simulink library "lib_EMachine_2017a"  (R2017b)
settings: Solver=VariableStepAuto  StartTime=0.0  StopTime=10.0  RelTol=1e-3
undefined symbols (not defined in the file): EngineTorqueReal, mot, motor_Trq, t_amb, time, tloop
libraries: simulink x5, autolibmappedmotor x3
(part 1 of 3)
settings Model: Creator=Di Russo  LastModifiedBy=Lyu19
settings CodeAppCC: StateflowObjectComments=on

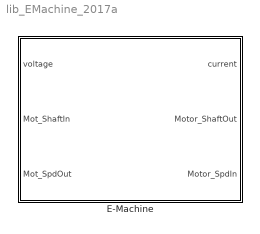
== system lib_EMachine_2017a ==
  E-Machine : Subsystem
      mask Display:
      | image('Images/motor.png')
      | color('red');
      | port_label('Input',1,'Volt');
      | port_label('Input',2,'ShaftIn');
      | port_label('Input',3,'SpdOut');
      | port_label('Output',1,'Crr');
      | port_label('Output',2,'ShaftOut');
      | port_label('Output',3,'SpdIn');

== system lib_EMachine_2017a/E-Machine ==
  voltage : Inport
  Mot_ShaftIn : Inport  Port=2
  Mot_SpdOut : Inport  Port=3
  Clutch Temporary 1 : Subsystem  Commented=on
  IMG Plant : Subsystem
      mask Display:
      | image('Images\Motor.png')
      | color('red');
      | port_label('Input',2,'Volt');
      | port_label('Input',3,'ShaftIn');
      | port_label('Input',4,'SpdOut');
      | port_label('Output',2,'Crr');
      | port_label('Output',3,'ShaftOut');
      | port_label('Output',4,'SpdIn');
  IMG Plant2 : Subsystem  Commented=on
      mask Display:
      | image('Images/motor.png')
      | color('red');
      | port_label('Input',2,'Volt');
      | port_label('Input',3,'SpdOut');
      | port_label('Input',1,'MCU_cmd');
      | port_label('Input',4,'ShaftIn');
      | port_label('Output',1,'Sensor_Out');
      | port_label('Output',2,'Crr');
      | port_label('Output',3,'MotTrqOut');
      | port_label('Output',4,'MotSpdIn');
  Soft MCU : Subsystem
      mask Display: image('SoftECU.jpg')
  current : Outport
  Motor_ShaftOut : Outport  Port=2
  Motor_SpdIn : Outport  Port=3
  tag scope: MCU_to_HCU=global
  wires:
  IMG Plant/4(SpdIn) -> Motor_SpdIn/1
  Mot_SpdOut/1 -> IMG Plant/4(SpdOut)
  Soft MCU/1(Out) -> [MCU_to_HCU]
  Soft MCU/2(Out1) -> IMG Plant/1("In1 ")  "MCU_to_Actuators"
  [HCU_to_HV_CAN] -> Soft MCU/1(In)
  IMG Plant/1(Out1) -> Soft MCU/2(In1)  "Sensors_to_MCU"
  Mot_ShaftIn/1 -> IMG Plant/3(MotShaftIn)
  IMG Plant/3(MotShaftOut) -> Motor_ShaftOut/1
  voltage/1 -> IMG Plant/2(voltage)
  IMG Plant/2(current) -> current/1

== system lib_EMachine_2017a/E-Machine/Clutch Temporary 1 ==
  In1 : Inport
  Constant : Constant  Value=0
  Memory : Memory
  Saturation : Saturate  UpperLimit=inf  LowerLimit=0
  Switch : Switch  Criteria=u2 > Threshold
  Out1 : Outport
  wires:
  Saturation/1 -> Memory/1
  Memory/1 -> Switch/1
  Constant/1 -> Switch/3
  In1/1 -> Saturation/1
  [cltch] -> Switch/2
  Switch/1 -> Out1/1

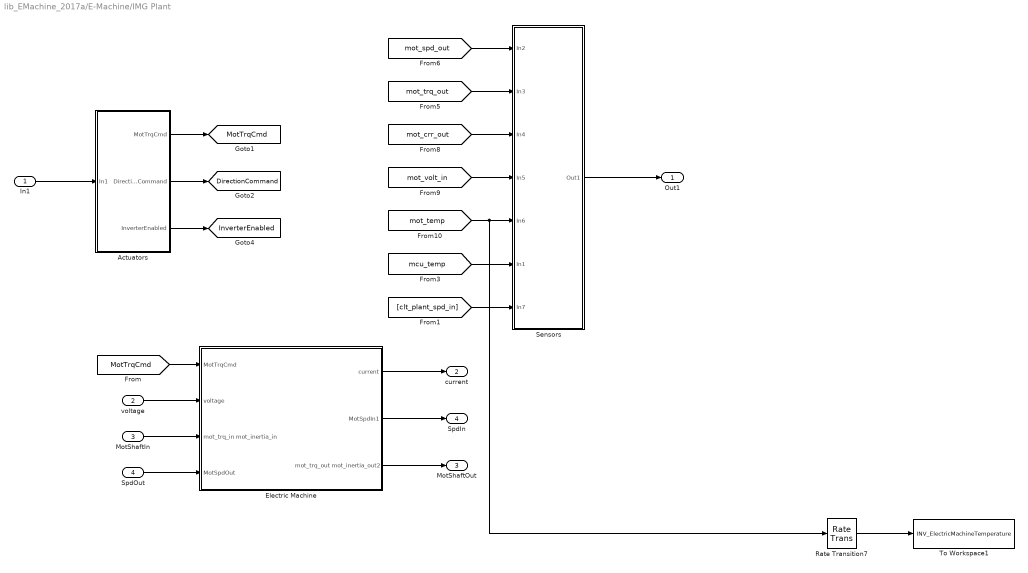
== system lib_EMachine_2017a/E-Machine/IMG Plant ==
  "In1 " : Inport
  voltage : Inport  Port=2
  MotShaftIn : Inport  Port=3
  SpdOut : Inport  Port=4
  " Actuators" : Subsystem
  Electric Machine : Subsystem
      mask Display:
      | image('Images\Motor.png')
      | color('red');
      | port_label('Input',1,'MotTrqCmd');
      | port_label('Input',2,'Volt');
      | port_label('Input',3,'ShaftIn');
      | port_label('Input',4,'SpdOut');
      | port_label('Output',1,'Crr')
      | port_label('Output',2,'SpdIn')
  Rate Transition7 : RateTransition  OutPortSampleTime=1
  Sensors : Subsystem
  To Workspace1 : ToWorkspace  VariableName=INV_ElectricMachineTemperature  SampleTime=-1
  Out1 : Outport
  current : Outport  Port=2
  MotShaftOut : Outport  Port=3
  SpdIn : Outport  Port=4
  tag scope: DirectionCommand=global, InverterEnabled=global, MotTrqCmd=global
  wires:
  [mot_spd_out] -> Sensors/1(In2)
  [clt_plant_spd_in] -> Sensors/7(In7)
  MotShaftIn/1 -> Electric Machine/3(mot_trq_in mot_inertia_in)
  SpdOut/1 -> Electric Machine/4(MotSpdOut)
  [mcu_temp] -> Sensors/6(In1)
  " Actuators"/3(InverterEnabled) -> [InverterEnabled]
  " Actuators"/2(DirectionCommand) -> [DirectionCommand]
  [mot_crr_out] -> Sensors/3(In4)
  "In1 "/1 -> " Actuators"/1(In1)
  [mot_volt_in] -> Sensors/4(In5)
  " Actuators"/1(MotTrqCmd) -> [MotTrqCmd]
  Sensors/1(Out1) -> Out1/1
  [mot_trq_out] -> Sensors/2(In3)
  Electric Machine/3(mot_trq_out mot_inertia_out2) -> MotShaftOut/1
  Electric Machine/2(MotSpdIn1) -> SpdIn/1
  Electric Machine/1(current) -> current/1
  [MotTrqCmd] -> Electric Machine/1(MotTrqCmd)
  voltage/1 -> Electric Machine/2(voltage)
  Rate Transition7/1 -> To Workspace1/1
  [mot_temp] -> Rate Transition7/1, Sensors/5(In6)

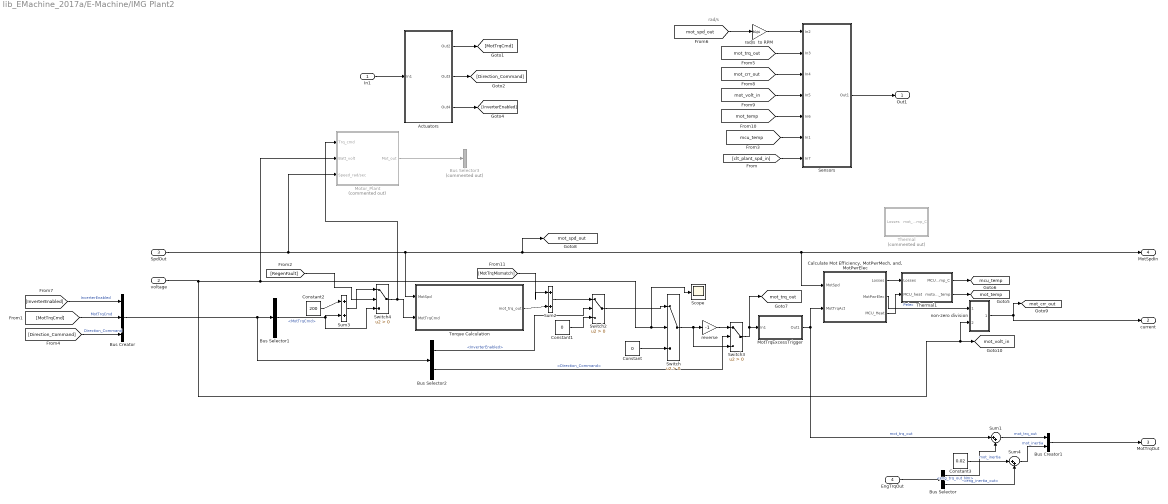
== system lib_EMachine_2017a/E-Machine/IMG Plant2 ==
  note: rad/s
  "In1 " : Inport
  voltage : Inport  Port=2
  SpdOut : Inport  Port=3
  EngTrqOut : Inport  Port=4
  " Actuators" : Subsystem
  Bus Creator : BusCreator  Inputs=3
  Bus Creator1 : BusCreator  Inputs=2
  Bus Selector : BusSelector  OutputSignals=eng_trq_out_Nm,eng_inertia_out
  Bus Selector1 : BusSelector  OutputSignals=MotTrqCmd
  Bus Selector2 : BusSelector  OutputSignals=InverterEnabled,Direction_Command
  Bus Selector3 : BusSelector  Commented=on  OutputSignals=Mot_current_A
  "Calculate Mot Efficiency, MotPwrMech, and, MotPwrElec" : Subsystem
  Constant : Constant  Value=0
  Constant1 : Constant  Value=0
  Constant2 : Constant  Value=200
  Constant3 : Constant  Value=0.02
  MotTrqExcessTrigger : Subsystem
  Motor_Plant : Subsystem  Commented=on
  Scope : Scope
  Sensors : Subsystem
  Sum{1..4} (4 alike) : Sum  Inputs=|++
  Switch{,2..4} (4 alike) : Switch  Criteria=u2 > Threshold
  Thermal : Subsystem  Commented=on
  Thermal1 : Subsystem
  Torque Calculation : Subsystem
  non-zero division : Subsystem
      mask Display: disp('divider \n I1/I2')
  rad/s  to RPM : Gain  Gain=30/pi
  reverse : Gain  Gain=-1
  Out1 : Outport
  current : Outport  Port=2
  MotTrqOut : Outport  Port=3
  MotSpdIn : Outport  Port=4
  tag scope: mcu_temp=global, mot_crr_out=global, mot_spd_out=global, mot_temp=global, mot_trq_out=global, mot_volt_in=global
  wires:
  [mot_temp] -> Sensors/5(In6)
  [mot_crr_out] -> Sensors/3(In4)
  "In1 "/1 -> " Actuators"/1(In1)
  [mot_volt_in] -> Sensors/4(In5)
  " Actuators"/1(Out2) -> [MotTrqCmd]
  Sensors/1(Out1) -> Out1/1
  [mot_trq_out] -> Sensors/2(In3)
  SpdOut/1 -> Motor_Plant/3(Speed_rad/sec), Torque Calculation/1(MotSpd), [mot_spd_out], MotSpdIn/1, "Calculate Mot Efficiency, MotPwrMech, and, MotPwrElec"/1(MotSpd)
  non-zero division/1(Out1) -> current/1, [mot_crr_out]
  [mcu_temp] -> Sensors/6(In1)
  [clt_plant_spd_in] -> Sensors/7(In7)
  " Actuators"/2(Out3) -> [Direction_Command]
  " Actuators"/3(Out4) -> [InverterEnabled]
  [Direction_Command] -> Bus Creator/3  "Direction_Command"
  [InverterEnabled] -> Bus Creator/1  "InverterEnabled"
  [MotTrqCmd] -> Bus Creator/2  "MotTrqCmd"
  [mot_spd_out] -> rad/s  to RPM/1
  rad/s  to RPM/1 -> Sensors/1(In2)
  Thermal1/1(MCU_temp_C) -> [mcu_temp]
  Constant2/1 -> Sum3/1
  Switch4/1 -> Motor_Plant/1(Trq_cmd), Torque Calculation/2(MotTrqCmd)
  Sum3/1 -> Switch4/1
  [RegenFault] -> Switch4/2
  Switch3/1 -> [mot_trq_out], MotTrqExcessTrigger/1(In1)
  reverse/1 -> Switch3/1
  Bus Selector2/2 -> Switch3/2  "<Direction_Command>"
  Switch2/1 -> Switch/1
  Constant1/1 -> Switch2/3
  Bus Selector2/1 -> Switch2/2  "<InverterEnabled>"
  Bus Selector1/1 -> Switch4/3, Sum3/2  "<MotTrqCmd>"
  Bus Creator/1 -> Bus Selector2/1, Bus Selector1/1
  Sum2/1 -> Switch2/1
  Torque Calculation/1(mot_trq_out) -> Sum2/2
  [MotTrqMismatch] -> Sum2/1
  Switch/1 -> Switch3/3, reverse/1
  Thermal1/2(motor_temp) -> [mot_temp]
  "Calculate Mot Efficiency, MotPwrMech, and, MotPwrElec"/3(MCU_Heat) -> Thermal1/2(MCU_heat)
  Constant/1 -> Switch/3
  "Calculate Mot Efficiency, MotPwrMech, and, MotPwrElec"/1(Losses) -> Thermal1/1(Losses)
  MotTrqExcessTrigger/1(Out1) -> Sum1/1, "Calculate Mot Efficiency, MotPwrMech, and, MotPwrElec"/2(MotTrqAct)  "mot_trq_out"
  "Calculate Mot Efficiency, MotPwrMech, and, MotPwrElec"/2(MotPwrElec) -> non-zero division/1(In1)  "Pelec"
  voltage/1 -> non-zero division/2(In2), [mot_volt_in], Motor_Plant/2(Batt_volt), Scope/1, Switch/2
  Bus Creator1/1 -> MotTrqOut/1
  Sum4/1 -> Bus Creator1/2  "mot_inertia"
  EngTrqOut/1 -> Bus Selector/1
  Sum1/1 -> Bus Creator1/1  "mot_trq_out"
  Bus Selector/2 -> Sum4/2  "<eng_inertia_out>"
  Constant3/1 -> Sum4/1  "mot_inertia"
  Bus Selector/1 -> Sum1/2  "<eng_trq_out_Nm>"
  Motor_Plant/1(Mot_out) -> Bus Selector3/1

== system lib_EMachine_2017a/E-Machine/Soft MCU ==
  In : Inport
  In1 : Inport  Port=2
  Bus Creator : BusCreator  Inputs=5
  Bus Creator1 : BusCreator  Inputs=2
  Bus Selector : BusSelector  OutputSignals=mot_spd_out,mot_trq_out,mot_volt_in
  Bus Selector1 : BusSelector  OutputSignals=M192_Command_Message.Inverter_Enable,M192_Command_Message.Torque_Command
  Constant : Constant  Value=0
  Data Type Conversion1 : DataTypeConversion
  Data Type Conversion2 : DataTypeConversion
  Data Type Conversion3 : DataTypeConversion
  ForwardDirection : Constant  Value=0
  Memory : Memory
  Subsystem : Subsystem
  Switch : Switch  Criteria=u2 ~= 0  Threshold=1
  Terminator : Terminator
  Torque Calculation1 : Subsystem  Commented=on
  Torque Calculation2 : Subsystem  Commented=on
  Torque Calculation3 : Subsystem
  diff_INV_state : MATLAB Function  TreatAsAtomicUnit=on
  diff_INV_state1 : MATLAB Function  TreatAsAtomicUnit=on
  Out : Outport
  Out1 : Outport  Port=2
  wires:
  Bus Selector1/2 -> Torque Calculation3/1(MotTrqReq)  "<Torque_Command>"
  Bus Selector/1 -> Torque Calculation3/2(MotSpd)  "<mot_spd_out>"
  Bus Selector/3 -> Torque Calculation3/4(Voltage)  "<mot_volt_in>"
  Torque Calculation3/1(current) -> Terminator/1
  Torque Calculation3/2(mot_trq_out1) -> Switch/1
  Subsystem/1(D3_Power_On_Timer) -> Bus Creator/4
  diff_INV_state1/1(y) -> Switch/2
  Bus Selector1/1 -> diff_INV_state/1(u), Memory/1  "<Inverter_Enable>"
  diff_INV_state/1(y) -> diff_INV_state1/1(u)
  ForwardDirection/1 -> Bus Creator/5  "Direction_Command"
  Data Type Conversion3/1 -> Bus Creator/1  "MotTrqCmd"
  Switch/1 -> Data Type Conversion3/1  "MotTrqCmd"
  Memory/1 -> Data Type Conversion1/1
  Data Type Conversion2/1 -> Bus Creator/3  "MotTrqFdbck"
  Bus Selector/2 -> Data Type Conversion2/1, Torque Calculation3/3(MotTrqFdbck)  "<mot_trq_out>"
  Data Type Conversion1/1 -> Bus Creator/2  "InverterEnabled"
  Constant/1 -> Switch/3
  Bus Creator/1 -> Out1/1, Bus Creator1/1  "MCU_to _Actuator"
  In/1 -> Bus Selector1/1  "HCU_to_MCU"
  Bus Creator1/1 -> Out/1  "MCU_CAN"
  In1/1 -> Bus Creator1/2, Bus Selector/1  "Sensors_to_MCU"

== system lib_EMachine_2017a/E-Machine/IMG Plant/ Actuators ==
  In1 : Inport
  Bus Selector : BusSelector  OutputSignals=MotTrqCmd,Direction_Command,InverterEnabled
  MotTrqCmd : Outport
  DirectionCommand : Outport  Port=2
  InverterEnabled : Outport  Port=3
  wires:
  Bus Selector/3 -> InverterEnabled/1  "<InverterEnabled>"
  Bus Selector/2 -> DirectionCommand/1  "<Direction_Command>"
  Bus Selector/1 -> MotTrqCmd/1  "<MotTrqCmd>"
  In1/1 -> Bus Selector/1

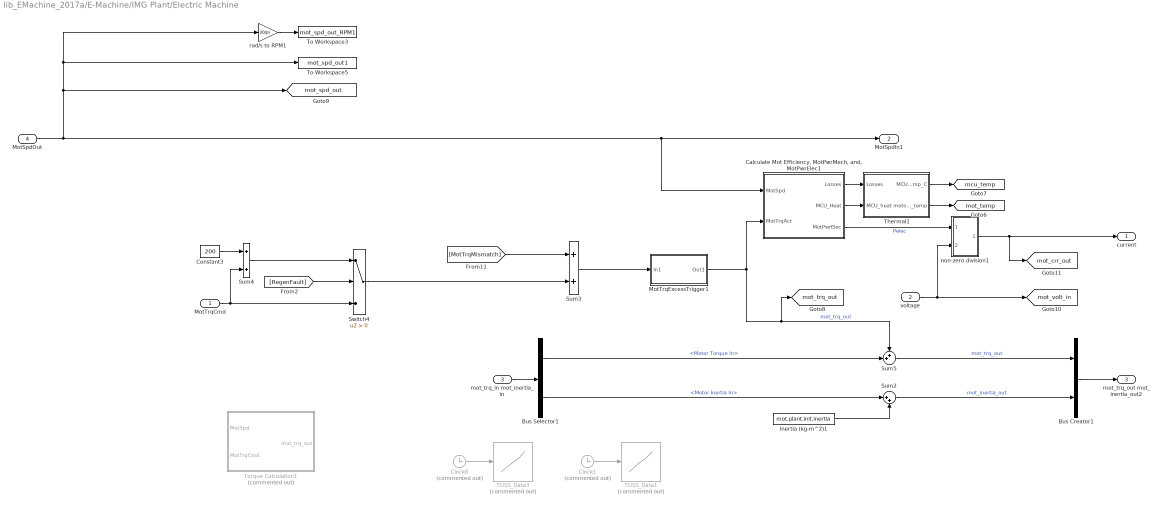
== system lib_EMachine_2017a/E-Machine/IMG Plant/Electric Machine ==
  MotTrqCmd : Inport
  voltage : Inport  Port=2
  mot_trq_in mot_inertia_in : Inport  Port=3
  MotSpdOut : Inport  Port=4
  Bus Creator1 : BusCreator  Inputs=2
  Bus Selector1 : BusSelector  OutputSignals=Motor Torque In,Motor Inertia In
  "Calculate Mot Efficiency, MotPwrMech, and, MotPwrElec1" : Subsystem
  Clock1 : Clock  Commented=on
  Clock8 : Clock  Commented=on
  Constant3 : Constant  Value=200
  Inertia (kg-m^2)1 : Constant  Value=mot.plant.init.inertia
  MotTrqExcessTrigger1 : Subsystem
  Sum2 : Sum  Inputs=|++
  Sum3 : Sum
  Sum4 : Sum
  Sum5 : Sum  Inputs=++|
  Switch4 : Switch  Criteria=u2 > Threshold
  TOSS_Data1 : Lookup_n-D  Commented=on  NumberOfTableDimensions=1  BreakpointsForDimension1=time  Table=EngineTorqueReal  InternalRulePriority=Speed  RndMeth=Simplest  InputSameDT=on
  TOSS_Data3 : Lookup_n-D  Commented=on  NumberOfTableDimensions=1  BreakpointsForDimension1=time  Table=motor_Trq  InternalRulePriority=Speed  RndMeth=Simplest  InputSameDT=on
  Thermal1 : Subsystem
  To Workspace3 : ToWorkspace  VariableName=mot_spd_out_RPM1  SampleTime=-1
      settings: Decimation=WORKSPACE_DECIMATION
  To Workspace5 : ToWorkspace  VariableName=mot_spd_out1  SampleTime=-1
      settings: Decimation=WORKSPACE_DECIMATION
  Torque Calculation1 : Subsystem  Commented=on
  non-zero division1 : Subsystem
      mask Display: disp('divider \n I1/I2')
  rad/s to RPM1 : Gain  Gain=30/pi
  current : Outport
  MotSpdIn1 : Outport  Port=2
  mot_trq_out mot_inertia_out2 : Outport  Port=3
  tag scope: mcu_temp=global, mot_crr_out=global, mot_spd_out=global, mot_temp=global, mot_trq_out=global, mot_volt_in=global
  wires:
  Clock1/1 -> TOSS_Data1/1
  Clock8/1 -> TOSS_Data3/1
  MotSpdOut/1 -> rad/s to RPM1/1, To Workspace5/1, [mot_spd_out], MotSpdIn1/1, "Calculate Mot Efficiency, MotPwrMech, and, MotPwrElec1"/1(MotSpd)
  rad/s to RPM1/1 -> To Workspace3/1
  Bus Selector1/1 -> Sum5/2  "<Motor Torque In>"
  Bus Selector1/2 -> Sum2/1  "<Motor Inertia In>"
  mot_trq_in mot_inertia_in/1 -> Bus Selector1/1
  Bus Creator1/1 -> mot_trq_out mot_inertia_out2/1
  Sum2/1 -> Bus Creator1/2  "mot_inertia_out"
  Inertia (kg-m^2)1/1 -> Sum2/2
  Sum5/1 -> Bus Creator1/1  "mot_trq_out"
  [MotTrqMismatch] -> Sum3/1
  voltage/1 -> [mot_volt_in], non-zero division1/2(In2)
  MotTrqCmd/1 -> Switch4/3, Sum4/2
  MotTrqExcessTrigger1/1(Out1) -> "Calculate Mot Efficiency, MotPwrMech, and, MotPwrElec1"/2(MotTrqAct), Sum5/1, [mot_trq_out]  "mot_trq_out"
  non-zero division1/1(Out1) -> current/1, [mot_crr_out]
  "Calculate Mot Efficiency, MotPwrMech, and, MotPwrElec1"/3(MotPwrElec) -> non-zero division1/1(In1)  "Pelec"
  Switch4/1 -> Sum3/2
  "Calculate Mot Efficiency, MotPwrMech, and, MotPwrElec1"/2(MCU_Heat) -> Thermal1/2(MCU_heat)
  Sum3/1 -> MotTrqExcessTrigger1/1(In1)
  Sum4/1 -> Switch4/1
  "Calculate Mot Efficiency, MotPwrMech, and, MotPwrElec1"/1(Losses) -> Thermal1/1(Losses)
  [RegenFault] -> Switch4/2
  Constant3/1 -> Sum4/1
  Thermal1/2(motor_temp) -> [mot_temp]
  Thermal1/1(MCU_temp_C) -> [mcu_temp]

== system lib_EMachine_2017a/E-Machine/IMG Plant/Sensors ==
  In2 : Inport
  In3 : Inport  Port=2
  In4 : Inport  Port=3
  In5 : Inport  Port=4
  In6 : Inport  Port=5
  In1 : Inport  Port=6
  In7 : Inport  Port=7
  Bus Creator : BusCreator  Inputs=7
  Out1 : Outport
  wires:
  In7/1 -> Bus Creator/7  "clt_plant_spd_in"
  In1/1 -> Bus Creator/6  "mcu_temp"
  In6/1 -> Bus Creator/5  "mot_temp"
  In3/1 -> Bus Creator/2  "mot_trq_out"
  In5/1 -> Bus Creator/4  "mot_volt_in"
  In4/1 -> Bus Creator/3  "mot_crr_out"
  In2/1 -> Bus Creator/1  "mot_spd_out"
  Bus Creator/1 -> Out1/1

== system lib_EMachine_2017a/E-Machine/IMG Plant2/ Actuators ==
  In1 : Inport
  Bus Selector : BusSelector  OutputSignals=MotTrqCmd,Direction_Command,InverterEnabled
  Out2 : Outport
  Out3 : Outport  Port=2
  Out4 : Outport  Port=3
  wires:
  Bus Selector/1 -> Out2/1  "<MotTrqCmd>"
  In1/1 -> Bus Selector/1
  Bus Selector/2 -> Out3/1  "<Direction_Command>"
  Bus Selector/3 -> Out4/1  "<InverterEnabled>"

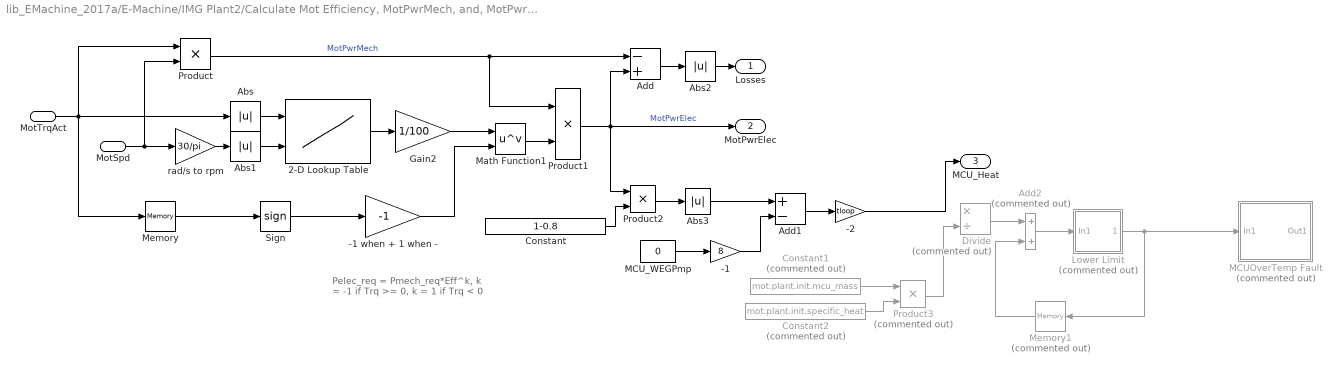
== system lib_EMachine_2017a/E-Machine/IMG Plant2/Calculate Mot Efficiency, MotPwrMech, and, MotPwrElec ==
  note: Pelec_req = Pmech_req*Eff^k,
      | k = -1 if Trq >= 0,
      | k = 1 if Trq < 0
  MotSpd : Inport
  MotTrqAct : Inport  Port=2
  -1 : Gain  Gain=8
  "-1 when + 1 when - " : Gain  Gain=-1
  -2 : Gain  Gain=tloop
  2-D Lookup Table : Lookup_n-D  BreakpointsForDimension1=mot.plant.init.eff_trq.idx2_trq  BreakpointsForDimension2=mot.plant.init.eff_trq.idx1_spd  Table=mot.plant.init.eff_trq.map  InternalRulePriority=Speed  RndMeth=Simplest  InputSameDT=on
  Abs{,1..3} (4 alike) : Abs
  Add : Sum  Inputs=-+
  Add1 : Sum  Inputs=+-
  Add2 : Sum  Commented=on
  Constant : Constant  Value=1-0.8
  Constant1 : Constant  Commented=on  Value=mot.plant.init.mcu_mass
  Constant2 : Constant  Commented=on  Value=mot.plant.init.specific_heat
  Divide : Product  Commented=on  Inputs=*/
  Gain2 : Gain  Gain=1/100
  Lower Limit : Subsystem  Commented=on  mask{Lolimit=t_amb+20}
      mask prompts: Lolimit "Lower Limit"
  MCUOverTemp Fault : Subsystem  Commented=on
  MCU_WEGPmp : Constant  Value=0
  Math Function1 : Math  Operator=pow  SaturateOnIntegerOverflow=on
  Memory : Memory
  Memory1 : Memory  Commented=on
  Product : Product
  Product1 : Product
  Product2 : Product
  Product3 : Product  Commented=on
  Sign : Signum
  rad/s to rpm : Gain  Gain=30/pi
  Losses : Outport
  MotPwrElec : Outport  Port=2
  MCU_Heat : Outport  Port=3
  wires:
  rad/s to rpm/1 -> Abs1/1
  Abs1/1 -> 2-D Lookup Table/2
  Sign/1 -> "-1 when + 1 when - "/1
  Abs/1 -> 2-D Lookup Table/1
  Gain2/1 -> Math Function1/1
  2-D Lookup Table/1 -> Gain2/1
  Product1/1 -> Product2/1, Add/2, MotPwrElec/1  "MotPwrElec"
  Product/1 -> Add/1, Product1/1  "MotPwrMech"
  MotTrqAct/1 -> Memory/1, Product/1, Abs/1
  MotSpd/1 -> Product/2, rad/s to rpm/1
  "-1 when + 1 when - "/1 -> Math Function1/2
  Abs2/1 -> Losses/1
  Add/1 -> Abs2/1
  Math Function1/1 -> Product1/2
  Memory/1 -> Sign/1
  Constant/1 -> Product2/2
  Product2/1 -> Abs3/1
  Abs3/1 -> Add1/1
  MCU_WEGPmp/1 -> -1/1
  Add1/1 -> -2/1
  -1/1 -> Add1/2
  -2/1 -> MCU_Heat/1
  Constant1/1 -> Product3/1
  Constant2/1 -> Product3/2
  Product3/1 -> Divide/2
  Divide/1 -> Add2/1
  Memory1/1 -> Add2/2
  Add2/1 -> Lower Limit/1(In1)
  Lower Limit/1(Out1) -> MCUOverTemp Fault/1(In1), Memory1/1

== system lib_EMachine_2017a/E-Machine/IMG Plant2/MotTrqExcessTrigger ==
  In1 : Inport
  Bias : Bias  Bias=55
  Bias1 : Bias  Bias=25
  Constant : Constant  Value=0
  Multiport Switch : MultiPortSwitch  DataPortOrder=Zero-based contiguous
  Out1 : Outport
  tag scope: MotTrqExcessTrig=global
  wires:
  Multiport Switch/1 -> Out1/1
  Bias/1 -> Multiport Switch/4
  In1/1 -> Multiport Switch/2, Bias/1, Bias1/1
  Bias1/1 -> Multiport Switch/3
  Constant/1 -> [MotTrqExcessTrig], Multiport Switch/1

== system lib_EMachine_2017a/E-Machine/IMG Plant2/Motor_Plant ==
  Trq_cmd : Inport
  Batt_volt : Inport  Port=2
  Speed_rad/sec : Inport  Port=3
  Add : Sum
  Bus Creator : BusCreator  Inputs=5
  Efficiency Calcs : Subsystem
  Memory : Memory
  Random Number : RandomNumber  Mean=0.1  Variance=0.1  SampleTime=0.01
  rad/sec to rpm : Gain  Gain=60/(2*3.14)
  Mot_out : Outport
  wires:
  Add/1 -> Memory/1
  Speed_rad/sec/1 -> rad/sec to rpm/1
  rad/sec to rpm/1 -> Bus Creator/2, Efficiency Calcs/1(Speed_rpm)  "Mot_spd_rpm"
  Random Number/1 -> Add/2
  Memory/1 -> Bus Creator/1, Efficiency Calcs/2(Torq_cmd_Nm)  "Mot_Trq_Nm"
  Bus Creator/1 -> Mot_out/1
  Trq_cmd/1 -> Add/1
  Batt_volt/1 -> Efficiency Calcs/3(Batt_volt)
  Efficiency Calcs/1(Mot_current) -> Bus Creator/3
  Efficiency Calcs/2(Mech_power_W) -> Bus Creator/4
  Efficiency Calcs/3(Elec_power_W) -> Bus Creator/5

== system lib_EMachine_2017a/E-Machine/IMG Plant2/Sensors ==
  In2 : Inport
  In3 : Inport  Port=2
  In4 : Inport  Port=3
  In5 : Inport  Port=4
  In6 : Inport  Port=5
  In1 : Inport  Port=6
  In7 : Inport  Port=7
  Bus Creator : BusCreator  Inputs=7
  Out1 : Outport
  wires:
  In6/1 -> Bus Creator/5  "mot_temp"
  In3/1 -> Bus Creator/2  "mot_trq_out"
  In5/1 -> Bus Creator/4  "mot_volt_in"
  In4/1 -> Bus Creator/3  "mot_crr_out"
  In2/1 -> Bus Creator/1  "mot_spd_out"
  Bus Creator/1 -> Out1/1
  In1/1 -> Bus Creator/6  "mcu_temp"
  In7/1 -> Bus Creator/7  "clt_plant_spd_in"

== system lib_EMachine_2017a/E-Machine/IMG Plant2/Thermal ==
  Losses : Inport
  Motor Thermal : Subsystem
  mot_temp_C : Outport
  wires:
  Losses/1 -> Motor Thermal/1(In1)  "[W]"
  Motor Thermal/1(Out1) -> mot_temp_C/1

== system lib_EMachine_2017a/E-Machine/IMG Plant2/Thermal1 ==
  Losses : Inport
  MCU_heat : Inport  Port=2
  MotInv_loop : Subsystem
  Motor Thermal : Subsystem  Commented=on
  MCU_temp_C : Outport
  motor_temp : Outport  Port=2
  wires:
  MCU_heat/1 -> MotInv_loop/2(In2)
  Losses/1 -> MotInv_loop/1(In1)  "[W]"
  MotInv_loop/1(Out1) -> MCU_temp_C/1
  MotInv_loop/2(Out2) -> motor_temp/1

== system lib_EMachine_2017a/E-Machine/IMG Plant2/Torque Calculation ==
  MotSpd : Inport
  MotTrqCmd : Inport  Port=2
  Abs : Abs
  Abs1 : Abs
  MinMax : MinMax  Inputs=2
  Product : Product
  Sign : Signum
  electric machine filter : Subsystem
  "max torque " : Subsystem
  mot_trq_out : Outport
  wires:
  "max torque "/1(max torque) -> Abs1/1
  MotSpd/1 -> "max torque "/2(speed)
  Sign/1 -> Product/1
  MinMax/1 -> Product/2
  Abs/1 -> MinMax/1
  Abs1/1 -> MinMax/2
  electric machine filter/1(filtered) -> mot_trq_out/1
  MotTrqCmd/1 -> "max torque "/1(cmd), Sign/1, Abs/1
  Product/1 -> electric machine filter/1(trq)

== system lib_EMachine_2017a/E-Machine/IMG Plant2/non-zero division ==
  note: original idea from Phil Sharer - ANL
      | original formula: u[1]\(u[2]+eps)*(u[2]!=0)
      | changes done by Gerald ZINI (dgey) - ANL (05\02\2001)
  note: (u[2]==0) is true then returns 1, thus (u[2]+(u[2]==0)) is equal to 0+1=1
  note: if u[2] == 0, then output == 0:
  note: (u[2]!=0) is false then returns 0
  note: and finally, the expression is: (u[1] \ 1) * 0 = 0
  note: (u[2]==0) is false then returns 0, thus (u[2]+(u[2]==0)) is equal to u[2]+0=u[2]
  note: if u[2] != 0, then output == u[1]\u[2]:
  note: (u[2]!=0) is true then returns 1
  note: and finally, the expression is: (u[1] \ u[2]) * 1 = u[1] \ u[2]
  In1 : Inport
  In2 : Inport  Port=2
  Fcn : Fcn  Expr=u[1]/(u[2]+(u[2]==0))*(u[2]!=0)
  Mux : Mux  Inputs=2
  Out1 : Outport
  wires:
  Mux/1 -> Fcn/1
  In1/1 -> Mux/1
  Fcn/1 -> Out1/1
  In2/1 -> Mux/2

== system lib_EMachine_2017a/E-Machine/Soft MCU/Subsystem ==
  MCU_RollingAliveCnt : Subsystem
  D3_Power_On_Timer : Outport
  wires:
  MCU_RollingAliveCnt/1(Out1) -> D3_Power_On_Timer/1  "D3_Power_On_Timer"

== system lib_EMachine_2017a/E-Machine/Soft MCU/Torque Calculation1 ==
  MotTrqReq : Inport
  MotSpd : Inport  Port=2
  MotTrqFdbck : Inport  Port=3
  Abs : Abs
  Abs1 : Abs
  MinMax : MinMax  Inputs=2
  Product : Product
  Sign : Signum
  "max torque " : Subsystem
  mot_trq_out : Outport
  wires:
  MotTrqFdbck/1 -> "max torque "/3(torque)
  Abs1/1 -> MinMax/2
  Abs/1 -> MinMax/1
  MinMax/1 -> Product/2
  Sign/1 -> Product/1
  MotTrqReq/1 -> Abs/1, Sign/1, "max torque "/1(Req)
  MotSpd/1 -> "max torque "/2(speed)
  "max torque "/1(max torque) -> Abs1/1
  Product/1 -> mot_trq_out/1

== system lib_EMachine_2017a/E-Machine/Soft MCU/Torque Calculation2 ==
  MotTrqReq : Inport
  MotSpd : Inport  Port=2
  MotTrqFdbck : Inport  Port=3
  mot_temp : Inport  Port=4
  mcu_temp : Inport  Port=5
  mot_volt_in : Inport  Port=6
  1-D Lookup Table : Lookup_n-D  NumberOfTableDimensions=1  BreakpointsForDimension1=[0,12600,12700,12800,12900,13000]  Table=[1,1,0.75,0.5,0.25,0]  InternalRulePriority=Speed  RndMeth=Simplest  InputSameDT=on
  1-D Lookup Table1 : Lookup_n-D  NumberOfTableDimensions=1  BreakpointsForDimension1=[0,410,415,420,425,430]  Table=[1,1,0.75,0.5,0.25,0]  InternalRulePriority=Speed  RndMeth=Simplest  InputSameDT=on
  1-D Lookup Table2 : Lookup_n-D  Commented=on  NumberOfTableDimensions=1  BreakpointsForDimension1=[0,90,100]  Table=[1,1,0]  InternalRulePriority=Speed  RndMeth=Simplest  InputSameDT=on
  1-D Lookup Table3 : Lookup_n-D  NumberOfTableDimensions=1  BreakpointsForDimension1=[0,150,170]  Table=[1,1,0]  InternalRulePriority=Speed  RndMeth=Simplest  InputSameDT=on
  Abs : Abs
  Abs1 : Abs
  Constant : Constant
  MinMax : MinMax  Inputs=2
  Product : Product
  Product1 : Product  Inputs=5
  Sign : Signum
  Terminator1 : Terminator
  "max torque " : Subsystem
  rad/s to RPM1 : Gain  Gain=30/pi
  mot_trq_out : Outport
  wires:
  1-D Lookup Table3/1 -> Product1/1
  Constant/1 -> Product1/2
  mcu_temp/1 -> Terminator1/1
  mot_temp/1 -> 1-D Lookup Table3/1
  1-D Lookup Table1/1 -> Product1/3
  mot_volt_in/1 -> 1-D Lookup Table1/1
  1-D Lookup Table/1 -> Product1/4
  Product1/1 -> mot_trq_out/1
  rad/s to RPM1/1 -> 1-D Lookup Table/1
  MotTrqFdbck/1 -> "max torque "/3(torque)
  Abs1/1 -> MinMax/2
  Abs/1 -> MinMax/1
  MinMax/1 -> Product/2
  Sign/1 -> Product/1
  MotTrqReq/1 -> Abs/1, Sign/1, "max torque "/1(Req)
  MotSpd/1 -> "max torque "/2(speed), rad/s to RPM1/1
  "max torque "/1(max torque) -> Abs1/1
  Product/1 -> Product1/5
